simulink model "sm_car_testrig_bus_VehBusChassisSpring"  (R2020a)
settings: Solver=VariableStepAuto  StartTime=0.0  StopTime=10.0  RelTol=1e-3
libraries: sm_car_lib x4, fl_lib x1, nesl_utility x1
Description:
  | Copyright 2020 The MathWorks, Inc.
settings Model: Creator=smiller  LastModifiedBy=smiller
settings DataIOCC: ReturnWorkspaceOutputs=off
settings DebuggingCC: ArithmeticOperatorsInVariantConditions=warning
settings SFSimCC: CustomCodeUndefinedFunction=UseInterfaceOnly

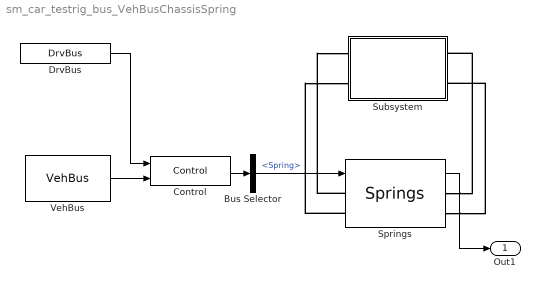
== system sm_car_testrig_bus_VehBusChassisSpring ==
  Bus Selector : BusSelector  OutputSignals=Chassis.Spring
  Control : sm_car_lib/Control/Control  popup_brake_control=Pedal  trq_ratio_front=1
      settings: AttributesFormatString=%<popup_brake_control>
  DrvBus : sm_car_lib/Inputs/DrvBus  SystemSampleTime=-1  Latency=0  AutoFrameSizeCalculation=off
  Springs : sm_car_lib/Springs Dampers/Springs  VariantControl=Variant1  LabelModeActiveChoice=Independent  Spring=Vehicle.Chassis.Spring  VariantLabel=Vehicle.Chassis.Spring.class.Value  InitTriggerDropdown=1
      settings: AttributesFormatString=%<ActiveVariant>
  Subsystem : Subsystem
  VehBus : sm_car_lib/Outputs/VehBus  SystemSampleTime=-1  Latency=0  AutoFrameSizeCalculation=off
  Out1 : Outport  OutDataTypeStr=Bus: VehicleChassisSpringBusDef  VectorParamsAs1DForOutWhenUnconnected=off
      settings: AttributesFormatString=%<OutDataTypeStr>
  wires:
  Springs/1 -> Out1/1
  Bus Selector/1 -> Springs/1  "<Spring>"
  Control/1 -> Bus Selector/1
  DrvBus/1 -> Control/1
  VehBus/1 -> Control/2
  connections:
  Springs/LConn1 -- Subsystem/LConn1
  Springs/LConn2 -- Subsystem/LConn2
  Springs/RConn1 -- Subsystem/RConn1
  Springs/RConn2 -- Subsystem/RConn2

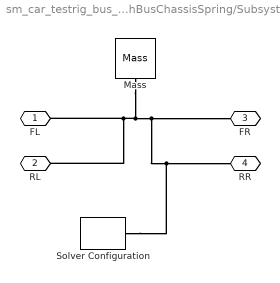
== system sm_car_testrig_bus_VehBusChassisSpring/Subsystem ==
  Mass : fl_lib/Mechanical/Translational Elements/Mass  mass=1 kg  v_specify=off  v_priority=High  v=0 m/s  v_nominal_specify=off  v_nominal_unit=m/s  v_nominal_value=1  f_specify=off  f_priority=None  f=0 N  f_nominal_specify=off  f_nominal_unit=N  f_nominal_value=1
  Solver Configuration : nesl_utility/Solver Configuration  PhysicalDomain=network_engine_domain  SubClassName=solver  LeftPortType=input  RightPortType=generic  Tones=[]  Harmonics=[]  SimulateNoise=off  Profile=off  UseLocalSampling=off  EnableSwitchedLinearOptims=on  FrequencyDomain=off  UseCCode=off  RelTol=0.001  AbsTol=1e-06  MinStep=1e-09  ToWorkspace=off  RevertToSquareIcSolve=off  NumHomotopyIterations=100  PhasorMode=off  PhasorModeNumHarmonics=1  DoDC=off  ResidualTolerance=1e-09  UseLocalSolver=off  LocalSolverChoice=NE_BACKWARD_EULER_ADVANCER  LocalSolverSampleTime=0.001  DoFixedCost=off  MaxNonlinIter=3  MaxModeIter=2  LinearAlgebra=auto  EquationFormulation=NE_TIME_EF  DelaysMemoryBudget=1024  AutomaticFiltering=on  FilteringTimeConstant=0.001  PartitionStorageMethod=AS_NEEDED  PartitionMemoryBudget=1024  PartitionMethod=FAST
  FL : PMIOPort  Side=Left
  RL : PMIOPort  Port=2  Side=Left
  FR : PMIOPort  Port=3  Side=Right
  RR : PMIOPort  Port=4  Side=Right
  connections:
  Mass/LConn1 -- Solver Configuration/RConn1 -- RR/RConn1 -- FR/RConn1 -- RL/RConn1 -- FL/RConn1
